simulink model "aircraft"  (R2024b)
settings: Solver=VariableStepAuto  StartTime=0.0  StopTime=1  RelTol=1e-3
undefined symbols (not defined in the file): Ad, Bd, Fd, x0
settings Model: Creator=Zoran Gaijc  LastModifiedBy=Zoran Gaijc

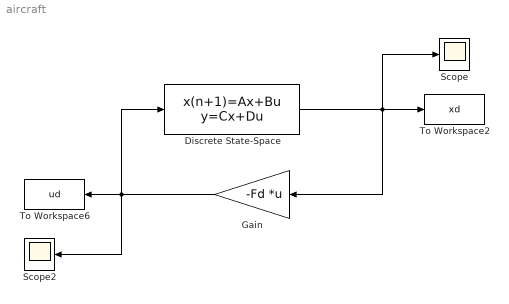
== system aircraft ==
  Discrete State-Space : DiscreteStateSpace  A=Ad  B=Bd  C=eye(5)  D=zeros(5,1)  InitialCondition=x0  SampleTime=-1
  Gain : Gain  Gain=-Fd  Multiplication=Matrix(K*u)
  Scope : Scope
  Scope2 : Scope
  To Workspace2 : ToWorkspace  VariableName=xd  SampleTime=-1
  To Workspace6 : ToWorkspace  VariableName=ud  SampleTime=-1
  wires:
  Gain/1 -> Scope2/1, To Workspace6/1, Discrete State-Space/1
  Discrete State-Space/1 -> Scope/1, To Workspace2/1, Gain/1
